simulink model "fisTRY"  (Simulink 7.7)
settings: Solver=ode45  StartTime=0.0  StopTime=120  FixedStep=Ts  RelTol=1e-3
values from neighbouring files (symbols this model uses):
  GCE = GE*(Kp-sqrt(Kp^2-4*Ki*Kd))/2/Ki    [fisTry.m]
  GCU = Ki/GE    [fisTry.m]
  GE = 10    [fisTry.m]
  GU = Kd/GCE    [fisTry.m]
  Ts = 0.1    [fisTry.m]
undefined symbols (not defined in the file or in its folder): DiscIntNeverNeededParam, Kd, Ki, Kp
libraries: simulink x2, cstblocks x2, fuzblock x1
settings Model: Creator=melanholly  LastModifiedBy=melanholly

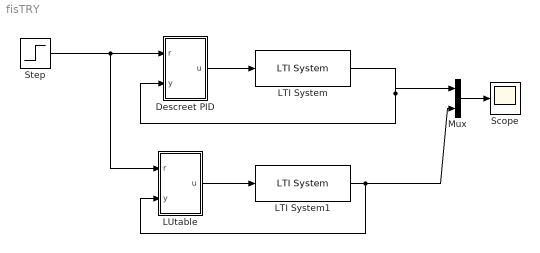
== system fisTRY ==
  Descreet PID : Subsystem
  LTI System : cstblocks/LTI System  SystemSampleTime=-1  sys=Plant  IC=[]
  LTI System1 : cstblocks/LTI System  SystemSampleTime=-1  sys=Plant  IC=[]
  LUtable : Subsystem
  Mux : Mux  Inputs=2
  Scope : Scope
      settings: TimeRange=12  YMin=0  YMax=1.223758865248227
  Step : Step  SampleTime=0
  wires:
  Descreet PID/1(u) -> LTI System/1
  Step/1 -> Descreet PID/1(r), LUtable/1(r)
  Mux/1 -> Scope/1
  LUtable/1(u) -> LTI System1/1
  LTI System1/1 -> Mux/2, LUtable/2(y)
  LTI System/1 -> Mux/1, Descreet PID/2(y)

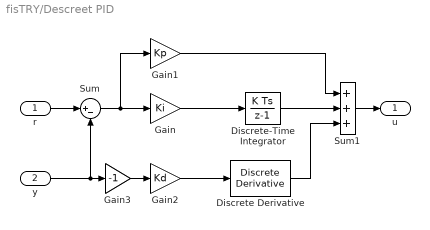
== system fisTRY/Descreet PID ==
  r : Inport
  y : Inport  Port=2
  Discrete Derivative : simulink/Discrete/Discrete Derivative  SystemSampleTime=-1  gainval=1.0  ICPrevScaledInput=0.0  OutMin=[]  OutMax=[]  OutDataType=fixdt(1, 16)  OutScaling=2^-10  DoSatur=off
  Discrete-Time Integrator : DiscreteIntegrator  SampleTime=Ts  ICPrevOutput=DiscIntNeverNeededParam  ICPrevScaledInput=DiscIntNeverNeededParam
  Gain : Gain  Gain=Ki  SampleTime=Ts
  Gain1 : Gain  Gain=Kp  SampleTime=Ts
  Gain2 : Gain  Gain=Kd  SampleTime=Ts
  Gain3 : Gain  Gain=-1  SampleTime=Ts
  Sum : Sum  Inputs=|+-
  Sum1 : Sum  Inputs=+++
  u : Outport
  wires:
  r/1 -> Sum/1
  y/1 -> Sum/2, Gain3/1
  Sum/1 -> Gain/1, Gain1/1
  Gain/1 -> Discrete-Time Integrator/1
  Sum1/1 -> u/1
  Gain1/1 -> Sum1/1
  Discrete-Time Integrator/1 -> Sum1/2
  Discrete Derivative/1 -> Sum1/3
  Gain2/1 -> Discrete Derivative/1
  Gain3/1 -> Gain2/1

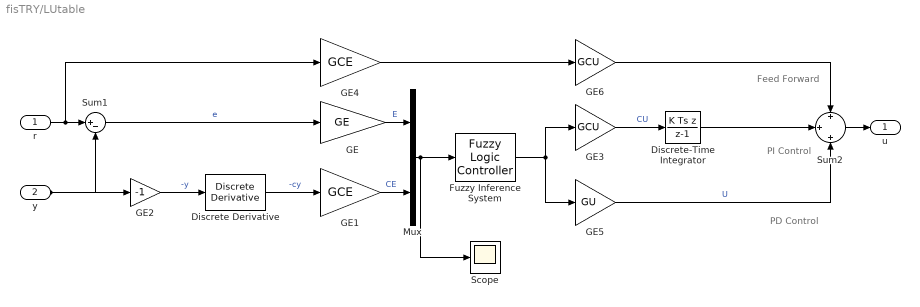
== system fisTRY/LUtable ==
  note: PD Control
  note: PI Control
  note: Feed Forward
  r : Inport
  y : Inport  Port=2
  Discrete Derivative : simulink/Discrete/Discrete Derivative  SystemSampleTime=-1  gainval=1  ICPrevScaledInput=0.0  OutMin=[]  OutMax=[]  OutDataType=fixdt(1, 16)  OutScaling=2^-10  DoSatur=off
  Discrete-Time Integrator : DiscreteIntegrator  IntegratorMethod=Integration: Backward Euler  SampleTime=Ts  ICPrevOutput=DiscIntNeverNeededParam  ICPrevScaledInput=DiscIntNeverNeededParam
  Fuzzy Inference System : fuzblock/Fuzzy Logic  Controller  SystemSampleTime=-1  fis=FIS
  GE : Gain  Gain=GE
  GE1 : Gain  Gain=GCE
  GE2 : Gain  Gain=-1
  GE3 : Gain  Gain=GCU
  GE4 : Gain  Gain=GCE
  GE5 : Gain  Gain=GU
  GE6 : Gain  Gain=GCU
  Mux : Mux  Inputs=2
  Scope : Scope
      settings: TimeRange=12  YMin=0  YMax=1.223758865248227
  Sum1 : Sum  Inputs=|+-
  Sum2 : Sum  Inputs=+|+|+
  u : Outport
  wires:
  Sum1/1 -> GE/1  "e"
  Mux/1 -> Fuzzy Inference System/1, Scope/1
  GE/1 -> Mux/1  "E"
  GE1/1 -> Mux/2  "CE"
  Fuzzy Inference System/1 -> GE3/1, GE5/1
  GE3/1 -> Discrete-Time Integrator/1  "CU"
  GE5/1 -> Sum2/3  "U"
  GE2/1 -> Discrete Derivative/1  "-y"
  Discrete Derivative/1 -> GE1/1  "-cy"
  r/1 -> Sum1/1, GE4/1
  y/1 -> Sum1/2, GE2/1
  Sum2/1 -> u/1
  GE4/1 -> GE6/1
  Discrete-Time Integrator/1 -> Sum2/2
  GE6/1 -> Sum2/1
